simulink model "lwdfa_1t_ssign"  (R2014b)
settings: Solver=ode45  StartTime=0.0  StopTime=10.0  RelTol=1e-3
settings Model: Creator=ravoson  LastModifiedBy=ravoson

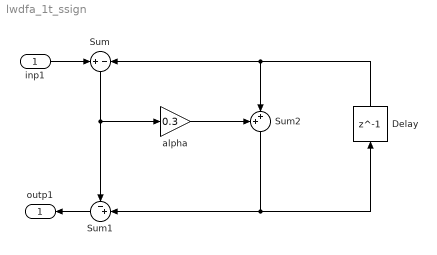
== system lwdfa_1t_ssign ==
  inp1 : Inport
  Delay : Delay  DelayLength=1  InitialCondition=0
  Sum : Sum  Inputs=+|-
  Sum1 : Sum  Inputs=-+|
  Sum2 : Sum  Inputs=++|
  alpha : Gain  Gain=0.3
  outp1 : Outport
  wires:
  inp1/1 -> Sum/1
  Sum1/1 -> outp1/1
  alpha/1 -> Sum2/1
  Sum2/1 -> Delay/1, Sum1/2
  Sum/1 -> alpha/1, Sum1/1
  Delay/1 -> Sum/2, Sum2/2
